simulink model "RW_control"  (R2016a)
settings: Solver=ode45  StartTime=0.0  StopTime=800  RelTol=1e-3
libraries: sim_operations x6
settings Model: Creator=Sanny  LastModifiedBy=Sanny
settings GRTTargetCC: GeneratePreprocessorConditionals=Use local settings

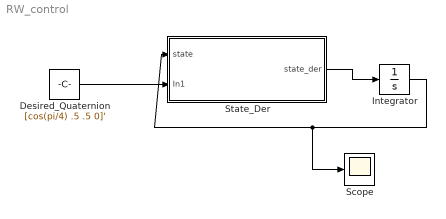
== system RW_control ==
  Desired_Quaternion : Constant  Value=[cos(pi/4) .5 .5 0]'
  Integrator : Integrator  InitialCondition=[1 0 0 0 0 0 0 0 0 0]'
  Scope : Scope
  State_Der : Subsystem  Description=State consists of quat, sat_ang_vel, wheel_ang_vels
  wires:
  State_Der/1(state_der) -> Integrator/1
  Integrator/1 -> Scope/1, State_Der/1(state)
  Desired_Quaternion/1 -> State_Der/2(In1)

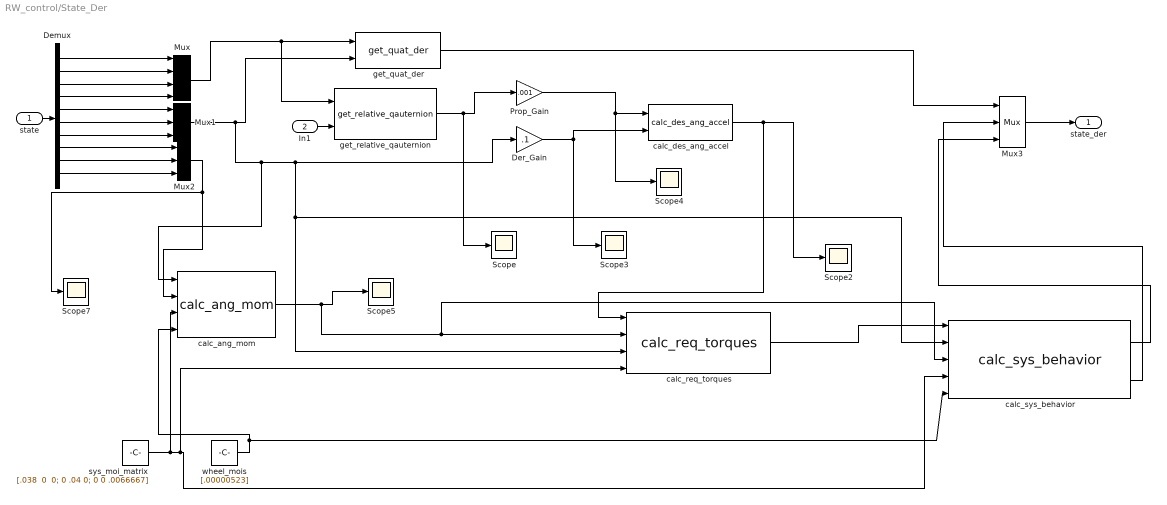
== system RW_control/State_Der ==
  state : Inport
  In1 : Inport  Port=2
  Demux : Demux  Outputs=10
  Der_Gain : Gain  Gain=.1
  Mux : Mux
  Mux1 : Mux  Inputs=3
  Mux2 : Mux  Inputs=3
  Mux3 : Mux  Inputs=3
  Prop_Gain : Gain  Gain=.001
  Scope{,2..5,7} (6 alike) : Scope
  calc_ang_mom : sim_operations/calc_ang_mom
  calc_des_ang_accel : sim_operations/calc_des_ang_accel
  calc_req_torques : sim_operations/calc_req_torques
  calc_sys_behavior : sim_operations/calc_sys_behavior
  get_quat_der : sim_operations/get_quat_der
  get_relative_qauternion : sim_operations/get_relative_qauternion
  sys_moi_matrix : Constant  Value="[.038  0  0; 0 .04 0; 0 0 .0066667]"
  wheel_mois : Constant  Value=[.00000523]
  state_der : Outport
  wires:
  state/1 -> Demux/1
  Demux/1 -> Mux/1
  Demux/2 -> Mux/2
  Demux/3 -> Mux/3
  Demux/4 -> Mux/4
  Demux/5 -> Mux1/1
  Demux/6 -> Mux1/2
  Demux/7 -> Mux1/3
  Demux/8 -> Mux2/1
  Demux/9 -> Mux2/2
  Demux/10 -> Mux2/3
  Mux/1 -> get_relative_qauternion/1, get_quat_der/1
  In1/1 -> get_relative_qauternion/2
  Prop_Gain/1 -> calc_des_ang_accel/1, Scope4/1
  Der_Gain/1 -> Scope3/1, calc_des_ang_accel/2
  calc_des_ang_accel/1 -> calc_req_torques/1, Scope2/1
  get_relative_qauternion/1 -> Scope/1, Prop_Gain/1
  get_quat_der/1 -> Mux3/1
  Mux3/1 -> state_der/1
  Mux1/1 -> calc_ang_mom/1, calc_sys_behavior/2, calc_req_torques/3, Der_Gain/1, get_quat_der/2
  sys_moi_matrix/1 -> calc_sys_behavior/4, calc_req_torques/4, calc_ang_mom/3
  Mux2/1 -> Scope7/1, calc_ang_mom/2
  wheel_mois/1 -> calc_sys_behavior/5, calc_ang_mom/4
  calc_ang_mom/1 -> calc_sys_behavior/3, calc_req_torques/2, Scope5/1
  calc_req_torques/1 -> calc_sys_behavior/1
  calc_sys_behavior/1 -> Mux3/3
  calc_sys_behavior/2 -> Mux3/2
